simulink model "lr4_2022"  (R2022a)
settings: Solver=ode23tb  StartTime=0.0  StopTime=0.5  MaxStep=1e-4  RelTol=1e-5
undefined symbols (not defined in the file): Const, DCsource, Eds, RL, UB
libraries: spsFourierLib x4, spsGroundLib x3, spsDCVoltageSourceLib x2, spsCurrentMeasurementLib x2, msbUtilities x2, spsVoltageMeasurementLib x2, spsSeriesRLCBranchLib x1, spsMultimeterLib x1, spsRMSLib x1, simulink x1, spsUniversalBridgeLib x1, spspowerguiLib x1
settings Model: Creator=Student11  LastModifiedBy=админ
settings SolverCC: AlgebraicLoopSolver=TrustRegion
settings DataIOCC: ReturnWorkspaceOutputs=off
settings DebuggingCC: ArithmeticOperatorsInVariantConditions=warning
settings SFSimCC: SimUseLocalCustomCode=off  CustomCodeUndefinedFunction=UseInterfaceOnly
settings RTWCC: RTWUseLocalCustomCode=off
settings CodeAppCC: StateflowObjectComments=on
settings SimscapeCC: SimscapeNormalizeSystem=off

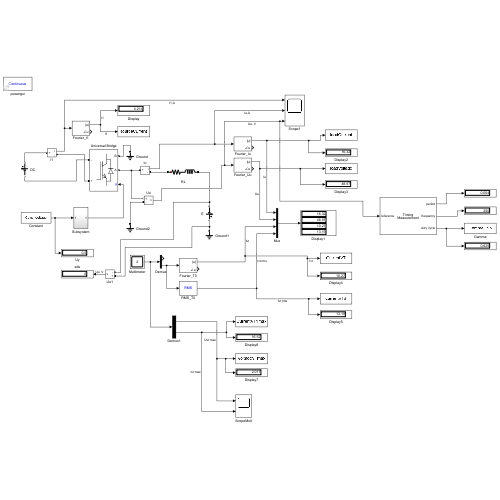
[thumbnail: Simulink's stored preview of the top-level diagram]
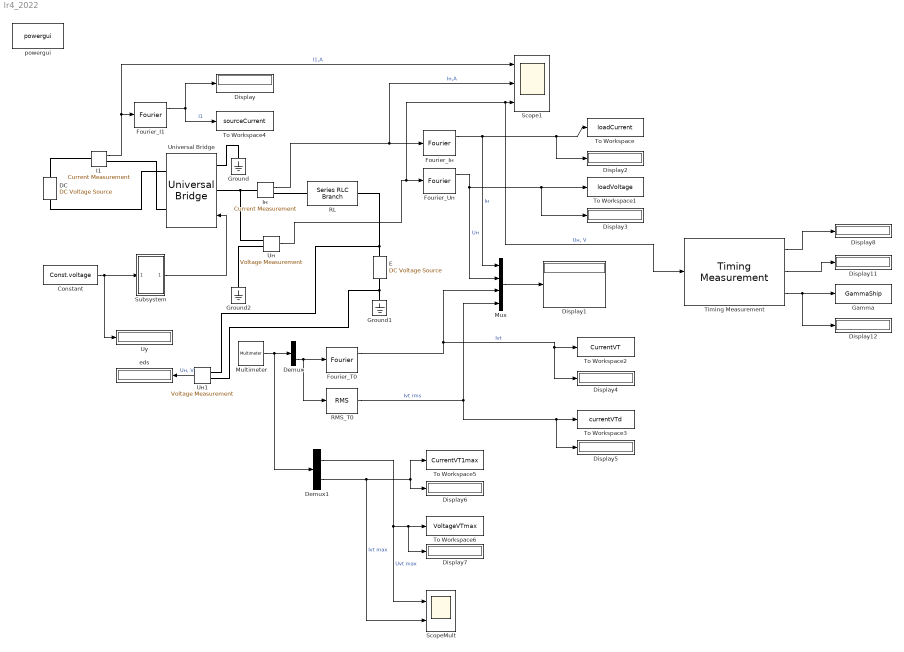
== system lr4_2022 ==
  " RL" : spsSeriesRLCBranchLib/Series RLC Branch  LConnTagsString=__new0  RConnTagsString=__new0  BranchType=RL  Resistance=RL.Res  Inductance=RL.Ind  SetiL0=off  InitialCurrent=0  Capacitance=1e-6  Setx0=off  InitialVoltage=0  Measurements=None
  Constant : Constant  Value=Const.voltage
  "DC " : spsDCVoltageSourceLib/DC Voltage Source  Amplitude=DCsource.Amplitude  Measurements=None
  Demux : Demux  Outputs=2
  Demux1 : Demux  Outputs=2
  Display{,1..8,11..12} (11 alike) : Display
  E : spsDCVoltageSourceLib/DC Voltage Source  Amplitude=Eds.voltage  Measurements=None
  Fourier_I1 : spsFourierLib/Fourier  Freq=Fourier.frec  n=Fourier.harmonic  InInit=[0, 0]  Ts=0
      settings: SourceProductBaseCode=PS
  Fourier_Iн : spsFourierLib/Fourier  Freq=Fourier.frec  n=Fourier.harmonic  InInit=[0, 0]  Ts=0
      settings: SourceProductBaseCode=PS
  Fourier_T0 : spsFourierLib/Fourier  Freq=Fourier.frec  n=Fourier.harmonic  InInit=[0, 0]  Ts=0
      settings: SourceProductBaseCode=PS
  Fourier_Uн : spsFourierLib/Fourier  Freq=Fourier.frec  n=Fourier.harmonic  InInit=[0, 0]  Ts=0
      settings: SourceProductBaseCode=PS
  Gamma : ToWorkspace  VariableName=GammaShip  SampleTime=-1
      settings: Save2DSignal=2-D array (concatenate along first dimension)
  Ground : spsGroundLib/Ground  LConnTagsString=a
  Ground1 : spsGroundLib/Ground  LConnTagsString=a
  Ground2 : spsGroundLib/Ground  LConnTagsString=a
  I1 : spsCurrentMeasurementLib/Current Measurement  PhasorSimulation=off  OutputType=Complex  PSBequivalent=0
  Iн : spsCurrentMeasurementLib/Current Measurement  PhasorSimulation=off  OutputType=Complex  PSBequivalent=0
  Multimeter : spsMultimeterLib/Multimeter  L=10  sel=[1 7]  yselected={}  Gain=[1 1]  OutputType=Complex  PlotAtSimulationStop=off  PhasorSimulation=off
  Mux : Mux
  RMS_T0 : spsRMSLib/RMS  TrueRMS=on  Freq=data.f  RMSInit=0  Ts=0
  Scope1 : Scope  NumInputPorts=3
  ScopeMult : Scope  NumInputPorts=2
  Subsystem : Subsystem
  Timing Measurement : msbUtilities/Timing Measurement  Period=on  Frequency=on  RiseTime=off  FallTime=off  DutyCycle=on  Delay=off  SameRefThreshold=on  GlobalRefThreshold=1  Range=[-1 1]  MeasurementType=80% / 20%  ThresholdMax=0.6  ThresholdMin=-0.6  DcRefThreshold=1  DelayRefThreshold=1  DelayTstThreshold=0
      settings: SourceProductBaseCode=AM
  To Workspace : ToWorkspace  VariableName=loadCurrent  SampleTime=-1
      settings: Save2DSignal=2-D array (concatenate along first dimension)
  To Workspace1 : ToWorkspace  VariableName=loadVoltage  SampleTime=-1
      settings: Save2DSignal=2-D array (concatenate along first dimension)
  To Workspace2 : ToWorkspace  VariableName=CurrentVT  SampleTime=-1
      settings: Save2DSignal=2-D array (concatenate along first dimension)
  To Workspace3 : ToWorkspace  VariableName=currentVTd  SampleTime=-1
      settings: Save2DSignal=2-D array (concatenate along first dimension)
  To Workspace4 : ToWorkspace  VariableName=sourceCurrent  SampleTime=-1
      settings: Save2DSignal=2-D array (concatenate along first dimension)
  To Workspace5 : ToWorkspace  VariableName=CurrentVT1max  SampleTime=-1
      settings: Save2DSignal=2-D array (concatenate along first dimension)
  To Workspace6 : ToWorkspace  VariableName=VoltageVTmax  SaveFormat=Timeseries  SampleTime=-1
      settings: Save2DSignal=2-D array (concatenate along first dimension)
  Universal Bridge : spsUniversalBridgeLib/Universal Bridge  Arms=2  SnubberResistance=UB.SnubberRs  SnubberCapacitance=UB.SnubberCs  Device=IGBT / Diodes  Ron=UB.R_on  Lon=0  ForwardVoltages="[UB.Vf  UB.Vfd]"  ForwardVoltage=0  GTOparameters=[ 10e-6 , 20e-6 ]  IGBTparameters=[ 1e-6 , 2e-6 ]  Measurements=All voltages and currents  Measurements_2=None  converterType=Rectifier
  Uн : spsVoltageMeasurementLib/Voltage Measurement  PhasorSimulation=off  OutputType=Complex  PSBequivalent=0
  Uн1 : spsVoltageMeasurementLib/Voltage Measurement  PhasorSimulation=off  OutputType=Complex  PSBequivalent=0
  Uу : Display
  eds : Display
  powergui : spspowerguiLib/powergui  Priority=1  SimulationMode=Continuous  SampleTime=50e-6  frequency=60  Iterations=50  frequencyindice=0  Pbase=100e6  ErrMax=1e-4  UnitsV=kV  UnitsW=MW  buscounter=0  FunctionMessages=off  echomessages=off  EnableUseOfTLC=off  CurrentSourceSwitches=off  DisableSnubberDevices=off  DisableRonSwitches=off  DisableVfSwitches=off  DisplayEquations=off  AutomaticDiscreteSolvers=off  SolverType=Tustin/Backward Euler (TBE)  Interpol=off  ExternalGateDelay=off  methode=off  Ts=100  x0status=blocks  SPID=on  SwTol=0  HookPort=off  NonlinearTolerance=1e-4  nMaxIteration=100  ContinueOnMaxIteration=off  RestoreLinks=warning  ResistiveCurrentMeasurement=off  Frange=[0:2:500]  Ylog=off  Xlog=on  ShowGrid=off  save=off  variable=ZData  structure=0  ZoomFFT=off  StartTime=0.0  cycles=1  DisplayStyle=1  fundamental=60  FreqAxis=off  MaxFrequency=1000  frequencyindicesteady=1  RmsSteady=1  display=off
  wires:
  I1/1 -> Scope1/1, Fourier_I1/1  "I1,A"
  Fourier_I1/1 -> To Workspace4/1, Display/1  "I1"
  Iн/1 -> Scope1/2, Fourier_Iн/1  "Iн,А"
  Uн/1 -> Timing Measurement/1, Scope1/3, Fourier_Uн/1  "Uн, V"
  Multimeter/1 -> Demux1/1, Demux/1
  Demux/2 -> RMS_T0/1, Fourier_T0/1
  Fourier_Iн/1 -> Mux/1, Display2/1, To Workspace/1  "Iн"
  Fourier_Uн/1 -> Display3/1, To Workspace1/1, Mux/2  "Uн"
  Fourier_T0/1 -> Mux/3, Display4/1, To Workspace2/1  "Ivt"
  RMS_T0/1 -> Display5/1, To Workspace3/1, Mux/4  "Ivt rms"
  Mux/1 -> Display1/1
  Constant/1 -> Subsystem/1(In1), Uу/1
  Subsystem/1(Out1) -> Universal Bridge/1
  Demux1/1 -> Display7/1, To Workspace6/1, ScopeMult/1  "Uvt max"
  Demux1/2 -> ScopeMult/2, Display6/1, To Workspace5/1  "Ivt max"
  Uн1/1 -> eds/1  "Uн, V"
  Timing Measurement/1 -> Display8/1
  Timing Measurement/2 -> Display11/1
  Timing Measurement/3 -> Gamma/1, Display12/1
  connections:
  Universal Bridge/LConn2 -- Ground/LConn1
  Iн/LConn1 -- Uн/LConn1 -- Universal Bridge/LConn1
  " RL"/RConn1 -- E/LConn1 -- Uн1/LConn2
  Ground1/LConn1 -- E/RConn1 -- Uн1/LConn1
  "DC "/RConn1 -- I1/LConn1
  I1/RConn1 -- Universal Bridge/RConn1
  "DC "/LConn1 -- Universal Bridge/RConn2
  " RL"/LConn1 -- Iн/RConn1
  Uн/LConn2 -- Ground2/LConn1

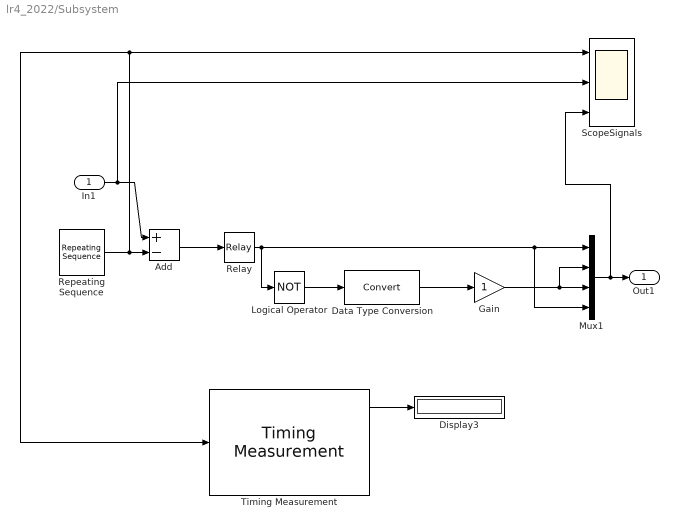
== system lr4_2022/Subsystem ==
  In1 : Inport
  Add : Sum  Inputs=+-
  Data Type Conversion : DataTypeConversion  SaturateOnIntegerOverflow=off  RndMeth=Floor
  Display3 : Display
  Gain : Gain
  Logical Operator : Logic  Operator=NOT  AllPortsSameDT=off  OutDataTypeStr=boolean
  Mux1 : Mux
  Relay : Relay  OffSwitchValue=0
  Repeating Sequence : simulink/Sources/Repeating Sequence  rep_seq_t=RepSec.Time  rep_seq_y=RepSec.Output
  ScopeSignals : Scope  NumInputPorts=3
  Timing Measurement : msbUtilities/Timing Measurement  Period=on  Frequency=on  RiseTime=off  FallTime=off  DutyCycle=on  Delay=off  SameRefThreshold=on  GlobalRefThreshold=1  Range=[-1 1]  MeasurementType=80% / 20%  ThresholdMax=0.6  ThresholdMin=-0.6  DcRefThreshold=1  DelayRefThreshold=1  DelayTstThreshold=0
      settings: SourceProductBaseCode=AM
  Out1 : Outport
  wires:
  In1/1 -> ScopeSignals/2, Add/1
  Mux1/1 -> ScopeSignals/3, Out1/1
  Repeating Sequence/1 -> Add/2, ScopeSignals/1, Timing Measurement/1
  Logical Operator/1 -> Data Type Conversion/1
  Add/1 -> Relay/1
  Gain/1 -> Mux1/3, Mux1/2
  Data Type Conversion/1 -> Gain/1
  Relay/1 -> Logical Operator/1, Mux1/1, Mux1/4
  Timing Measurement/1 -> Display3/1
